simulink model "simSchemeGPSKalmanFilter"  (R2021a)
settings: Solver=FixedStepAuto  StartTime=0.0  StopTime=250  FixedStep=T_s  RelTol=1e-3
values from neighbouring files (symbols this model uses):
  K1 = W1 / X    [LPVGainScheduling.m]
  K2 = W2 / X    [LPVGainScheduling.m]
  K3 = W3 / X    [LPVGainScheduling.m]
  K4 = W4 / X    [LPVGainScheduling.m]
  T_s = 0.1    [main.m]
  x0 = [-30;0;0]    [main.m]
settings Model: PacingRate=1000  Creator=nicol  LastModifiedBy=nicol

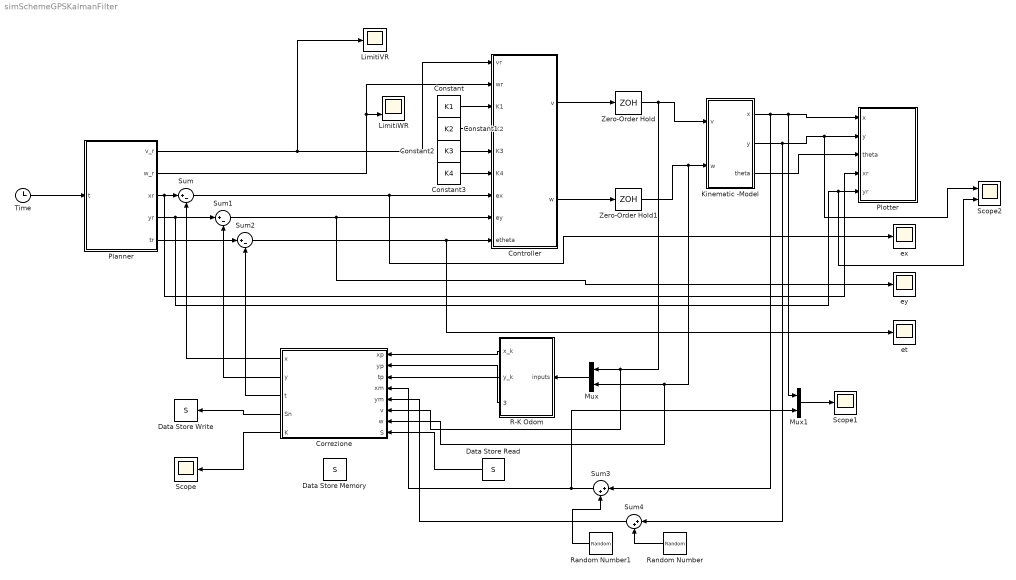
== system simSchemeGPSKalmanFilter ==
  Constant : Constant  Value=K1
  Constant1 : Constant  Value=K2
  Constant2 : Constant  Value=K3
  Constant3 : Constant  Value=K4
  Controller : MATLAB Function  TreatAsAtomicUnit=on
  Correzione : MATLAB Function  TreatAsAtomicUnit=on
  Data Store Memory : DataStoreMemory  DataStoreName=S  ReadBeforeWriteMsg=warning  WriteAfterWriteMsg=warning  WriteAfterReadMsg=warning  InitialValue=eye(3)  ShowAdditionalParam=off
  Data Store Read : DataStoreRead  DataStoreName=S  IndexOptions=Index vector (dialog)  Indices=1  OutputSizes=1
  Data Store Write : DataStoreWrite  DataStoreName=S  IndexOptions=Index vector (dialog)  Indices=1  OutputSizes=1
  Kinematic -Model : Subsystem
  LimitiVR : Scope
  LimitiWR : Scope  NumInputPorts=2
  Mux : Mux  Inputs=2
  Mux1 : Mux  Inputs=2
  Planner : MATLAB Function  TreatAsAtomicUnit=on
  Plotter : MATLAB Function  TreatAsAtomicUnit=on
  R-K Odom : Subsystem
  Random Number : RandomNumber  Variance=0.001  SampleTime=T_s
  Random Number1 : RandomNumber  Variance=0.001  SampleTime=T_s
  Scope : Scope
  Scope1 : Scope
  Scope2 : Scope  NumInputPorts=2
  Sum : Sum  Inputs=|+-
  Sum1 : Sum  Inputs=|+-
  Sum2 : Sum  Inputs=|+-
  Sum3 : Sum  Inputs=|++
  Sum4 : Sum  Inputs=|++
  Time : Clock
  Zero-Order Hold : ZeroOrderHold  SampleTime=T_s
  Zero-Order Hold1 : ZeroOrderHold  SampleTime=T_s
  et : Scope
  ex : Scope
  ey : Scope
  wires:
  Time/1 -> Planner/1(t)
  Planner/3(xr) -> Sum/1, Plotter/4(xr)
  Planner/4(yr) -> Scope2/2, Plotter/5(yr), Sum1/1
  Planner/5(tr) -> Sum2/1
  Sum2/1 -> et/1, Controller/9(etheta)
  Sum/1 -> ex/1, Controller/7(ex)
  Planner/2(w_r) -> Controller/2(wr), LimitiWR/2
  Constant/1 -> Controller/3(K1)
  Constant1/1 -> Controller/4(K2)
  Constant2/1 -> Controller/5(K3)
  Constant3/1 -> Controller/6(K4)
  Sum1/1 -> ey/1, Controller/8(ey)
  Planner/1(v_r) -> LimitiVR/1, Controller/1(vr)
  Mux1/1 -> Scope1/1
  Correzione/5(K) -> Scope/1
  Sum3/1 -> Mux1/2, Correzione/4(xm)
  R-K Odom/1(x_k) -> Correzione/1(xp)
  R-K Odom/2(y_k) -> Correzione/2(yp)
  Mux/1 -> R-K Odom/1(inputs)
  Data Store Read/1 -> Correzione/8(S)
  Correzione/4(Sn) -> Data Store Write/1
  R-K Odom/3(theta_k) -> Correzione/3(tp)
  Sum4/1 -> Correzione/5(ym)
  Correzione/1(x) -> Sum/2
  Correzione/2(y) -> Sum1/2
  Correzione/3(t) -> Sum2/2
  Kinematic -Model/3(theta) -> Plotter/3(theta)
  Kinematic -Model/2(y) -> Sum4/1, Scope2/1, Plotter/2(y)
  Kinematic -Model/1(x) -> Sum3/1, Mux1/1, Plotter/1(x)
  Random Number/1 -> Sum4/2
  Random Number1/1 -> Sum3/2
  Controller/1(v) -> Zero-Order Hold/1
  Controller/2(w) -> Zero-Order Hold1/1
  Zero-Order Hold1/1 -> Correzione/7(w), Mux/2, Kinematic -Model/2(w)
  Zero-Order Hold/1 -> Correzione/6(v), Mux/1, Kinematic -Model/1(v)

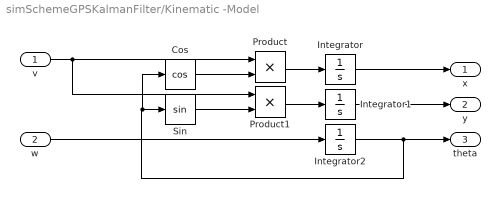
== system simSchemeGPSKalmanFilter/Kinematic -Model ==
  v : Inport
  w : Inport  Port=2
  Cos : Trigonometry  Operator=cos
  Integrator : Integrator  InitialCondition=x0(1)
  Integrator1 : Integrator  InitialCondition=x0(2)
  Integrator2 : Integrator  InitialCondition=x0(3)
  Product : Product
  Product1 : Product
  Sin : Trigonometry
  x : Outport
  y : Outport  Port=2
  theta : Outport  Port=3
  wires:
  v/1 -> Product1/1, Product/1
  Integrator2/1 -> theta/1, Cos/1, Sin/1
  Sin/1 -> Product1/2
  Integrator/1 -> x/1
  w/1 -> Integrator2/1
  Product1/1 -> Integrator1/1
  Integrator1/1 -> y/1
  Product/1 -> Integrator/1
  Cos/1 -> Product/2

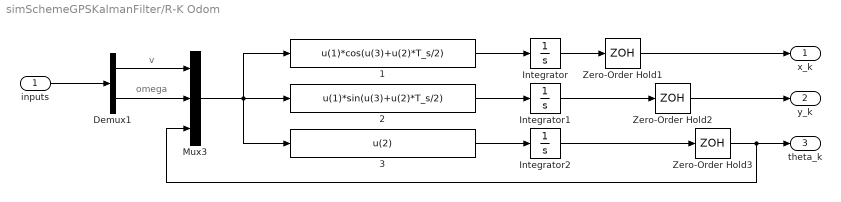
== system simSchemeGPSKalmanFilter/R-K Odom ==
  note: omega
  note: v
  inputs : Inport
  " 1" : Fcn  Expr=u(1)*cos(u(3)+u(2)*T_s/2)
  " 2" : Fcn  Expr=u(1)*sin(u(3)+u(2)*T_s/2)
  " 3" : Fcn  Expr=u(2)
  Demux1 : Demux  Outputs=2
  Integrator : Integrator  InitialCondition=x0(1)
  Integrator1 : Integrator  InitialCondition=x0(2)
  Integrator2 : Integrator  InitialCondition=x0(3)
  Mux3 : Mux  Inputs=3
  Zero-Order Hold1 : ZeroOrderHold  SampleTime=T_s
  Zero-Order Hold2 : ZeroOrderHold  SampleTime=T_s
  Zero-Order Hold3 : ZeroOrderHold  SampleTime=T_s
  x_k : Outport
  y_k : Outport  Port=2
  theta_k : Outport  Port=3
  wires:
  " 1"/1 -> Integrator/1
  " 2"/1 -> Integrator1/1
  Mux3/1 -> " 3"/1, " 1"/1, " 2"/1
  " 3"/1 -> Integrator2/1
  Integrator/1 -> Zero-Order Hold1/1
  Integrator1/1 -> Zero-Order Hold2/1
  Zero-Order Hold3/1 -> Mux3/3, theta_k/1
  Zero-Order Hold2/1 -> y_k/1
  Zero-Order Hold1/1 -> x_k/1
  Demux1/1 -> Mux3/1
  Demux1/2 -> Mux3/2
  inputs/1 -> Demux1/1
  Integrator2/1 -> Zero-Order Hold3/1

== matlab function simSchemeGPSKalmanFilter/Planner ==
  data: t input; v_r output; w_r output; xr output; yr output; tr output
function [v_r,w_r,xr,yr,tr] = getTraj(t)
A =5;
w = 0.1;
% if(t >= 60 && t <= 150)
%     A = 0.93;
% elseif(t>150 && t <= 210)
%     A = 0.80;
% elseif(t > 210)
%     A = 0.85;
% end
% definizione ingressi sfruttando la piattezza differenziale
xr    =   t;
yr    =   A*sin(w*t)+A*sin(2*w*t);
% derivata prima
x_d   =   1;
y_d   =   A*cos(w*t)*w+2*A*cos(2*w*t)*w;
tr    = atan2(y_d,x_d);
% derivata seconda
x_dd =  0;
y_dd =  -A*sin(w*t)*w*w-4*A*sin(2*w*t)*w*w;
% definizione ingressi corrispondenti
v_r  = sqrt(x_d*x_d + y_d*y_d);
w_r  = (y_dd*x_d - x_dd*y_d)/(x_d*x_d + y_d*y_d);
end

== matlab function simSchemeGPSKalmanFilter/Plotter ==
  settings: updateMethod=DISCRETE
  data: x input; y input; theta input; xr input; yr input
function plotDD(x,y,theta,xr,yr)
persistent xp yp xrr yrr
if(isempty(xp))
    xp  = [];
    yp  = [];
    xrr = [];
    yrr = [];
end
% Definizione Parametri Strutturali Robot
W = 2;                    % Base triangolo
H = 1.7;                  % Altezza triangolo
coder.extrinsic("patch");
% Definizione Robot -> Struttura Geometrica : Triangolo
vertici_triangolo  = [-W/2 W/2 -W/2; 
                      -H/2  0  +H/2;
                        0   0    0];
% Defizione Matrice in SO(3) -> Rotazione Rispetto all'asse z
R = [cos(theta) ,   -sin(theta) , 0;
     sin(theta) ,  cos(theta) , 0;
         0      ,       0     , 1];
% Rotazione Dei Vettori Posizione Vertici Differential Drive
rotazione   = R*vertici_triangolo;
% Traslazione
traslazione = [x , x , x;
               y , y , y;
               0 , 0 , 0];
% memorizzazione
xp  = [xp , x];
yp  = [yp , y];
xrr = [xrr , xr];
yrr = [yrr , yr];
% Posa := Traslazione + Rotazione
posa        = traslazione + rotazione;
% Apertura Finestra Di Disegno
clf;
hold on;
grid on;
axis square;
% xlim([-100, 350]);
% ylim([-100, 350]);
% Rappresentazione Robot
patch([posa(1,:)],[posa(2,:)],[posa(3,:)],'r');
plot(xp,yp,'b--');
plot(xrr,yrr,'r--');

end

== matlab function simSchemeGPSKalmanFilter/Correzione ==
  data: x output; xp input; y output; yp input; tp input; xm input; ym input; v input; w input; t output; S input; Sn output; K output
function [x,y,t,Sn,K]= fcn(xp,yp,tp,xm,ym,v,w,S)
% Sampling Time
T_s = 0.1;
% Definizione Innovazione
e                = [xp;yp] - [xm;ym];
% Calcolo Jacobiano 
Gt                =       [1 , 0 , -v*T_s*sin(tp+(w*T_s/2));
                          0 , 1 ,  v*T_s*cos(tp+(w*T_s/2));
                          0 , 0 ,            1           ];
% Covarianza Rumore Processo e Misura
Rt                =0.3   *[1.0000    0.0000    0.0000;
                          0.0000    1.0000    0.0000;
                          0.0000    0.0000    1.0000];
Qt                =0.001 *[1.000    0.000;
                           0.000    1.000];
% Definizione Matrice Covarianze
Ss               = Gt*S*Gt' + Rt;
% Calcolo Guadagno di Kalman
Ht                = [1 0 0;0 1 0];
K                = Ss*Ht'*inv(Ht*Ss*Ht' + Qt);
% Correzione
x                = xp + K(1,:)*e;
y                = yp + K(2,:)*e;
t                = tp + K(3,:)*e;
Sn               = (eye(3) - K*Ht)*Ss*(eye(3)-K*Ht)'+K*Qt*K';
end

== matlab function simSchemeGPSKalmanFilter/Controller ==
  data: v output; w output; vr input; wr input; K1 input; K2 input; K3 input; K4 input; ex input; ey input; etheta input
function [v,w] = control(vr,wr,K1,K2,K3,K4,ex,ey,etheta)
% definizione limiti 
vMin =    1;
vMax =    5;
wMin =   -5;
wMax =    5;
% Controllo Gain Scheduling
p1   = ((vr-vMin)/(vMax-vMin))*((wr -wMin)/(wMax - wMin));
p2   = ((vr - vMin)/(vMax-vMin))*((wMax-wr)/(wMax - wMin));
p3   = ((vMax-vr)/(vMax-vMin))*((wMax-wr)/(wMax -wMin));
p4   = ((vMax-vr)/(vMax-vMin))*((wr -wMin)/(wMax -wMin));
% Guadagno Controllore Gain Scheduling
K    = p1*K1+p2*K2+p3*K3+p4*K4;
% Definizione ingressi Addizionali
u1   = K(1,1)*ex+K(1,2)*ey+K(1,3)*etheta;
u2   = K(2,1)*ex+K(2,2)*ey+K(2,3)*etheta;
% Ingressi Effettivi
v    = vr*cos(etheta)-u1;
w    = wr - u2;
end
